simulink library "ayazLiftingBody_cl"  (R2018b)
settings: Solver=VariableStepAuto  StartTime=0.0  StopTime=10.0  RelTol=1e-3
undefined symbols (not defined in the file or in its folder): ini_euler_ang, ini_O_Vcm_o, ini_OwB, ini_Rcm_o
libraries: thrAttachPtKinematics_ul x3, eulAng2RotMat_ul x1
settings Model: Creator=mcobb  LastModifiedBy=mcobb

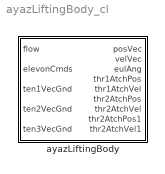
== system ayazLiftingBody_cl ==
  ayazLiftingBody : Subsystem

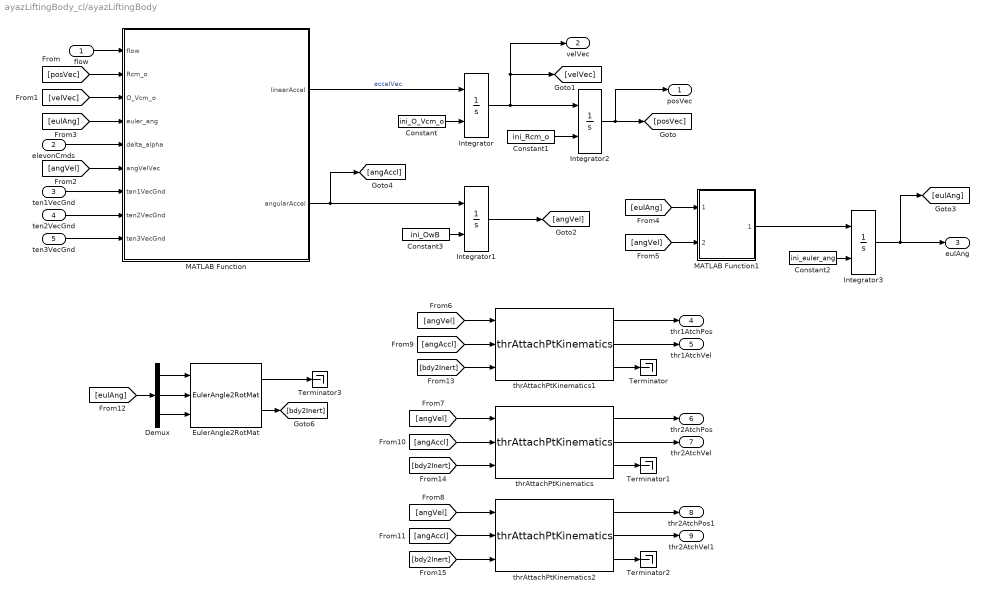
== system ayazLiftingBody_cl/ayazLiftingBody ==
  flow : Inport
  elevonCmds : Inport  Port=2
  ten1VecGnd : Inport  Port=3
  ten2VecGnd : Inport  Port=4
  ten3VecGnd : Inport  Port=5
  Constant : Constant  Value=ini_O_Vcm_o
  Constant1 : Constant  Value=ini_Rcm_o
  Constant2 : Constant  Value=ini_euler_ang
  Constant3 : Constant  Value=ini_OwB
  Demux : Demux  Outputs=3
  EulerAngle2RotMat : eulAng2RotMat_ul/EulerAngle2RotMat  SystemSampleTime=-1
  Integrator{,1..3} (4 alike) : Integrator  InitialConditionSource=external
  MATLAB Function : MATLAB Function  TreatAsAtomicUnit=on
  MATLAB Function1 : MATLAB Function  TreatAsAtomicUnit=on
  Terminator{,1..3} (4 alike) : Terminator
  thrAttachPtKinematics : thrAttachPtKinematics_ul/thrAttachPtKinematics  theAtchPosVec=sim_param.tether_imp_nodes.R2n_cm
  thrAttachPtKinematics1 : thrAttachPtKinematics_ul/thrAttachPtKinematics  theAtchPosVec=sim_param.tether_imp_nodes.R1n_cm
  thrAttachPtKinematics2 : thrAttachPtKinematics_ul/thrAttachPtKinematics  theAtchPosVec=sim_param.tether_imp_nodes.R3n_cm
  "posVec " : Outport
  velVec : Outport  Port=2
  eulAng : Outport  Port=3
  thr1AtchPos : Outport  Port=4
  thr1AtchVel : Outport  Port=5
  thr2AtchPos : Outport  Port=6
  thr2AtchVel : Outport  Port=7
  thr2AtchPos1 : Outport  Port=8
  thr2AtchVel1 : Outport  Port=9
  wires:
  ten3VecGnd/1 -> MATLAB Function/9(ten3VecGnd)
  ten2VecGnd/1 -> MATLAB Function/8(ten2VecGnd)
  ten1VecGnd/1 -> MATLAB Function/7(ten1VecGnd)
  [eulAng] -> MATLAB Function/4(euler_ang)
  [angVel] -> MATLAB Function/6(angVelVec)
  Integrator3/1 -> eulAng/1, [eulAng]
  [velVec] -> MATLAB Function/3(O_Vcm_o)
  [posVec] -> MATLAB Function/2(Rcm_o)
  Integrator2/1 -> "posVec "/1, [posVec]
  Integrator/1 -> velVec/1, [velVec], Integrator2/1
  Integrator1/1 -> [angVel]
  MATLAB Function/2(angularAccel) -> [angAccl], Integrator1/1
  MATLAB Function/1(linearAccel) -> Integrator/1  "accelVec"
  flow/1 -> MATLAB Function/1(flow)
  elevonCmds/1 -> MATLAB Function/5(delta_alpha)
  Constant/1 -> Integrator/2
  Constant1/1 -> Integrator2/2
  Constant2/1 -> Integrator3/2
  Constant3/1 -> Integrator1/2
  [eulAng] -> MATLAB Function1/1(eulAng)
  [angVel] -> MATLAB Function1/2(angVel)
  MATLAB Function1/1(eulAngDeriv) -> Integrator3/1
  [angVel] -> thrAttachPtKinematics1/1
  [angVel] -> thrAttachPtKinematics/1
  [angVel] -> thrAttachPtKinematics2/1
  [angAccl] -> thrAttachPtKinematics1/2
  [angAccl] -> thrAttachPtKinematics/2
  [angAccl] -> thrAttachPtKinematics2/2
  [eulAng] -> Demux/1
  Demux/2 -> EulerAngle2RotMat/2
  Demux/1 -> EulerAngle2RotMat/1
  Demux/3 -> EulerAngle2RotMat/3
  EulerAngle2RotMat/2 -> [bdy2Inert]
  [bdy2Inert] -> thrAttachPtKinematics1/3
  [bdy2Inert] -> thrAttachPtKinematics/3
  [bdy2Inert] -> thrAttachPtKinematics2/3
  thrAttachPtKinematics1/1 -> thr1AtchPos/1
  thrAttachPtKinematics/1 -> thr2AtchPos/1
  thrAttachPtKinematics2/1 -> thr2AtchPos1/1
  thrAttachPtKinematics1/2 -> thr1AtchVel/1
  thrAttachPtKinematics/2 -> thr2AtchVel/1
  thrAttachPtKinematics1/3 -> Terminator/1
  thrAttachPtKinematics/3 -> Terminator1/1
  thrAttachPtKinematics2/2 -> thr2AtchVel1/1
  thrAttachPtKinematics2/3 -> Terminator2/1
  EulerAngle2RotMat/1 -> Terminator3/1

== matlab function ayazLiftingBody_cl/ayazLiftingBody/MATLAB Function ==
  data: sim_param parameter; flow input; linearAccel output size=[3 1]; Rcm_o input; O_Vcm_o input; euler_ang input; delta_alpha input; angVelVec input; angularAccel output size=[3 1]; ten1VecGnd input; ten2VecGnd input; ten3VecGnd input
function [linearAccel, angularAccel] = B_F_and_T_aero(sim_param,flow,Rcm_o,...
    O_Vcm_o,euler_ang,delta_alpha,angVelVec,ten1VecGnd,ten2VecGnd,...
    ten3VecGnd)

% %% extract from structure
% aero_param = sim_param.aero_param;
% env_param = sim_param.env_param;
% turbine_param = sim_param.turbine_param;
% elevons_param = sim_param.elevons_param;
% 
% CM_nom = elevons_param.CM_nom;
% k_CM = elevons_param.k_CM;
% 
% MI = sim_param.geom_param.MI;
% Ixx = MI(1,1);
% Iyy = MI(2,2);
% Izz = MI(3,3);
% Izz_added = sim_param.geom_param.Izz_added;
% 
% Rcb_cm = sim_param.geom_param.center_of_buoy;
% 
% R1n_cm = sim_param.tether_imp_nodes.R1n_cm;
% R2n_cm = sim_param.tether_imp_nodes.R2n_cm;
% R3n_cm = sim_param.tether_imp_nodes.R3n_cm;
% 
% % buoyancy force in the ko direction
% fz_buoy = sim_param.geom_param.F_buoy;
% 
% % buoyancy force in the O frame
% O_F_buoy = [0;0;fz_buoy];
% 
% 
% % R11_g = sim_param.tether_imp_nodes.R11_g;
% % R21_g = sim_param.tether_imp_nodes.R21_g;
% % R31_g = sim_param.tether_imp_nodes.R31_g;
% 
m = sim_param.geom_param.mass;
m_added = sim_param.geom_param.m_added;
% 
% rho = env_param.density;
% 
% span = sim_param.geom_param.span;
% chord = sim_param.geom_param.chord;
% AR = sim_param.geom_param.AR;
% Rmidspan_cm = [0;span/4;0];
% 
% Sref = aero_param.Sref;
% 
% pcl_mw = aero_param.pcl_mw;
% pcd_mw = aero_param.pcd_mw;
% pcm_mw = aero_param.pcm_mw;
% 
% HS_Sref = aero_param.HS_Sref;
% VS_Sref = aero_param.VS_Sref;
% pcl_VS = aero_param.pcl_VS;
% pcd_VS = aero_param.pcd_VS;
% pcm_VS = aero_param.pcm_VS;
% 
% A_turbine = turbine_param.A_turbine;
% CD_turb = turbine_param.CD_turb;
% Cp_turb = turbine_param.Cp_turb;
% 
% % position vectors
% Rac_cm = sim_param.geom_param.aero_center;
% Rvs_cm = aero_param.Rvs_cm;
% R1turb_cm = turbine_param.R1turb_cm;
% R2turb_cm = turbine_param.R2turb_cm;
% 
% % change in effective angle of attack due to control surfaces
% delta_alp1 = delta_alpha(1);
% delta_alp2 = delta_alpha(2);
% 
% % delta elevator control
% delta_pitch = (1/2)*(delta_alp1 + delta_alp2);
% delta_roll = delta_alp1 - delta_alp2;
% 
% % rotation matrix
% [oCb,bCo] = rotation_sequence(euler_ang);
% 
% % relative velocity in O frame
% O_Vrel = flow - O_Vcm_o;
% 
% % relative/apparent velocity in the B frame
% B_Vrel = bCo*O_Vrel;
% 
% % breaking down the relative velocity in the B frame
% vxb = B_Vrel(1); vyb = B_Vrel(2); vzb = B_Vrel(3);
% 
% % apparent flow velocity in the XZ plane
% V_app_xz = sqrt(vxb^2 + vzb^2);
% 
% % apparent flow velocity in the Xy plane
% V_app_xy = sqrt(vxb^2 + vyb^2);
% 
% % angle of attack and side slip angle
% alpha = atan2(vzb,vxb);
% beta = asin(vyb/norm(B_Vrel));
% 
% % converting to degree
% alpha_deg = alpha*(180/pi);
% beta_deg = beta*(180/pi);
% 
% %% IMPORTANT
% % limiting alpha values
% if norm(alpha_deg) > 29
%     CL_mw = polyval(pcl_mw,29);
%     CD_mw = polyval(pcd_mw,29) + CL_mw^2/(pi*AR);
%     CM_mw = polyval(pcm_mw,alpha_deg);
%     
% else
%     CL_mw = polyval(pcl_mw,alpha_deg);
%     CD_mw = polyval(pcd_mw,alpha_deg) + CL_mw^2/(pi*AR);
%     CM_mw = polyval(pcm_mw,alpha_deg);
%     
% end
% 
% % limiting beta values
% if norm(beta_deg) > 29
%     
%     CL_VS = polyval(pcl_VS,29);
%     CD_VS = polyval(pcd_VS,29);
%     CM_VS = polyval(pcm_VS,beta_deg);
%     
% else
%     CL_VS = polyval(pcl_VS,beta_deg);
%     CD_VS = polyval(pcd_VS,beta_deg);
%     CM_VS = polyval(pcm_VS,beta_deg);
%     
% end
% 
% %% MAIN WING FORCES
% % dynamic pressure
% dyn_press = (1/2)*rho*norm(B_Vrel)^2;
% 
% % wing force
% Fd_mw_app = CD_mw*dyn_press*Sref;
% Fl_mw_app = CL_mw*dyn_press*Sref;
% 
% % HS force
% Fd_hs_app = CD_mw*dyn_press*HS_Sref;
% Fl_hs_app = CL_mw*dyn_press*HS_Sref;
% 
% % drag direction
% mw_drag_dir = B_Vrel/norm(B_Vrel);
% 
% % lift direction
% mw_lz = sqrt(1/(1 + (vzb/vxb)^2));
% mw_lx = -mw_lz*(vzb/vxb);
% mw_lift_dir = [mw_lx;0;mw_lz];
% 
% % aerodynamic forces on main wing in the body frame
% B_F_drag_mw = (Fd_mw_app + Fd_hs_app)*mw_drag_dir;
% B_F_lift_mw = (Fl_mw_app + Fl_hs_app)*mw_lift_dir;
% 
% B_F_aero_mw = B_F_drag_mw + B_F_lift_mw;
% 
% %% VERTICAL STABILIZER FORCES
% % aerodynamic forces in the apparent flow frame
% Fd_VS_app = CD_VS*dyn_press*VS_Sref;
% Fl_VS_app = CL_VS*dyn_press*VS_Sref;
% 
% % lift direction
% vs_ly = sqrt(1/(1 + (vyb/vxb)^2));
% vs_lx = -vs_ly*(vyb/vxb);
% vs_lift_dir = [vs_lx;vs_ly;0];
% 
% % aerodynamic forces on rudder in the body frame
% B_F_drag_VS = Fd_VS_app*mw_drag_dir;
% B_F_lift_VS = Fl_VS_app*vs_lift_dir;
% 
% B_F_aero_VS = B_F_drag_VS + B_F_lift_VS;
% 
% %% TURBINE FORCES
% 
% Fd_turb1 = CD_turb*dyn_press*A_turbine;
% Fd_turb2 = CD_turb*dyn_press*A_turbine;
% 
% B_F_turb1 = Fd_turb1*mw_drag_dir;
% B_F_turb2 = Fd_turb2*mw_drag_dir;
% 
% gen_power = 2*0.5*rho*(vxb^3)*Cp_turb*A_turbine;
% 
% if gen_power < 0
%     gen_power = 0;
% elseif norm(gen_power) > turbine_param.rated_power
%     gen_power = turbine_param.rated_power;
% end
% 
% %% TORQUES
% % torque about roll axis due to aileron
% T_roll = [(CM_nom*k_CM*delta_roll)*dyn_press*Sref*chord;0;0];
% 
% % torque about pitch axis due to aileron
% T_pitch = [0;(CM_nom*k_CM*delta_pitch)*dyn_press*Sref*chord;0];
% 
% % torque due to aero forces on main wing about CM in the B frame
% B_T_aero_mw = cross(Rac_cm,B_F_aero_mw) + T_roll + T_pitch;
% 
% % torque due to aero forces on main wing about CM in the B frame
% B_T_aero_VS = cross(Rvs_cm,B_F_aero_VS);
% 
% % torque due to turbine drag
% B_T_aero_turb = cross(R1turb_cm,B_F_turb1) + cross(R2turb_cm,B_F_turb2);
% 
% B_F_aero = B_F_turb1 + B_F_turb2 + B_F_drag_VS + B_F_lift_VS + Fd_VS_app + Fl_VS_app + B_F_aero_mw;
% 
% % torque due to the three tethers in the B frame
% B_Tt1 = cross(R1n_cm,(bCo*ten1VecGnd(:)));
% B_Tt2 = cross(R2n_cm,(bCo*ten2VecGnd(:)));
% B_Tt3 = cross(R3n_cm,(bCo*ten3VecGnd(:)));
% 
% F_buoy = bCo*[0;0;sim_param.geom_param.vol*sim_param.env_param.density*sim_param.env_param.grav];
% 
% % torque due to buoyancy about CM in the B frame
% B_T_buoy = cross(Rcb_cm,(bCo*O_F_buoy));
% 
% % torque due to gravity about CM
% B_T_grav = [0;0;0];
% 
% F_grav = [0;0;-m*sim_param.env_param.grav];
% 
% B_F_Net = B_F_aero + F_grav + F_buoy + bCo*ten1VecGnd(:) + bCo*ten2VecGnd(:) + bCo*ten3VecGnd(:);
% 
% 
% mass_matrix = [1/(m+m_added(1)) 0 0;0 1/(m+m_added(2)) 0;0 0 1/(m+m_added(3))];
%% extracting values from sim parameters structure
N = sim_param.N;

env_param = sim_param.env_param;
geom_param = sim_param.geom_param;
aero_param = sim_param.aero_param;
turbine_param = sim_param.turbine_param;
tether_param = sim_param.tether_param;
tether_imp_nodes = sim_param.tether_imp_nodes;


m = geom_param.mass;
g = env_param.grav;
rho = env_param.density;

CD_cylinder = tether_param.CD_cylinder;
tether_youngs = tether_param.tether_youngs;


Rcb_cm = geom_param.center_of_buoy;
Rac_cm = geom_param.aero_center;
R1turb_cm = turbine_param.R1turb_cm;
R2turb_cm = turbine_param.R2turb_cm;


Rvs_cm = aero_param.Rvs_cm;

R1n_cm = tether_imp_nodes.R1n_cm;
R2n_cm = tether_imp_nodes.R2n_cm;
R3n_cm = tether_imp_nodes.R3n_cm;

R11_g = tether_imp_nodes.R11_g;
R21_g = tether_imp_nodes.R21_g;
R31_g = tether_imp_nodes.R31_g;


% calculate tether masses and spring stiffness
tether_density = tether_param.tether_density;
tether_dia = tether_param.tether_diameter;
zeta = tether_param.damping_ratio;

% tether_masses = ((tether_density*(pi/4)).*tether_dia.^2).*unstretched_l;

%% spring stiffness
% tether_CS = (pi/4)*tether_dia.^2;
% 
% full_length_stiff = tether_youngs*(tether_CS.*[1/unstretched_l(1);1/unstretched_l(2);1/unstretched_l(3)]);
% 
% ks1 = full_length_stiff(1)*(N-1);
% ks2 = full_length_stiff(2)*(N-1);
% ks3 = full_length_stiff(3)*(N-1);

%% damping coeff
% full length damping coeff
% full_length_d_coeff = zeta*(2*sqrt(full_length_stiff*m));

% tether damping coeff
% damping_coeff = full_length_d_coeff*(N-1);

% c1 = damping_coeff(1);
% c2 = damping_coeff(2);
% c3 = damping_coeff(3);


%% rotations
[oCb,bCo] = rotation_sequence(euler_ang);
% platform
% pCo = [cos(plat_ang) sin(plat_ang) 0; -sin(plat_ang) cos(plat_ang) 0; 0 0 1];
% oCp = pCo';


% L1 = unstretched_l(1);
% L2 = unstretched_l(2);
% L3 = unstretched_l(3);
% 
% L1i = L1/(N-1);
% L2i = L2/(N-1);
% L3i = L3/(N-1);


%% force calculations
% buoyancy force in the ko direction
fz_buoy = geom_param.F_buoy;

% buoyancy force in the O frame
O_F_buoy = [0;0;fz_buoy];

% gravity force in the ko direction
fz_grav = -m*g;

% gravity force in the O frame
O_F_grav = [0;0;fz_grav];

% calculate aerodynamic forces on the lifting body
aero_F = B_F_and_T_aero(sim_param,flow,Rcm_o,O_Vcm_o,euler_ang,delta_alpha);

B_F_aero_mw = aero_F.B_F_aero_mw;
B_F_aero_VS = aero_F.B_F_aero_VS;
B_F_turb1 = aero_F.B_F_turb1;
B_F_turb2 = aero_F.B_F_turb2;

B_T_aero_mw = aero_F.B_T_aero_mw;
B_T_aero_VS = aero_F.B_T_aero_VS;
B_T_aero_turb = aero_F.B_T_aero_turb;


O_F_aero_mw = oCb*B_F_aero_mw;
O_F_aero_VS = oCb*B_F_aero_VS;
O_F_turb1 = oCb*B_F_turb1;
O_F_turb2 = oCb*B_F_turb2;

% %% forces acting on the center of mass
O_F_ext = O_F_buoy + O_F_grav + O_F_aero_mw + O_F_aero_VS + O_F_turb1 + O_F_turb2 +...
    ten1VecGnd + ten2VecGnd + ten3VecGnd;

mass_matrix = [1/(m+m_added(1)) 0 0;0 1/(m+m_added(2)) 0;0 0 1/(m+m_added(3))];


linearAccel = oCb*(mass_matrix*bCo*O_F_ext);
B_T_buoy = cross(Rcb_cm,(bCo*O_F_buoy));
% torque due to gravity about CM
B_T_grav = [0;0;0];


% torque due to the three tethers in the B frame
B_Tt1 = cross(R1n_cm,(bCo*ten1VecGnd));
B_Tt2 = cross(R2n_cm,(bCo*ten2VecGnd));
B_Tt3 = cross(R3n_cm,(bCo*ten3VecGnd));

B_T_ext = B_T_buoy + B_T_grav + B_T_aero_mw + B_T_aero_VS + B_T_aero_turb + ...
    B_Tt1 + B_Tt2 + B_Tt3;

Tx = B_T_ext(1);
Ty = B_T_ext(2);
Tz = B_T_ext(3);

wx = angVelVec(1);
wy = angVelVec(2);
wz = angVelVec(3);

MI = sim_param.geom_param.MI;
Ixx = MI(1,1);
Iyy = MI(2,2);
Izz = MI(3,3);
Izz_added = sim_param.geom_param.Izz_added;

angularAccel = [...
    (1/Ixx)*(Tx + (Iyy - Izz)*wy*wz);...
    (1/Iyy)*(Ty + (Izz - Ixx)*wx*wz);...
    (1/(Izz+Izz_added))*(Tz + (Ixx - Iyy)*wx*wy)];

end

== matlab function ayazLiftingBody_cl/ayazLiftingBody/MATLAB Function1 ==
  data: eulAng input; eulAngDeriv output; angVel input
function eulAngDeriv = fcn(eulAng,angVel)

wx = angVel(1);
wy = angVel(2);
wz = angVel(3);

ph = eulAng(1);
th = eulAng(2);

eulAngDeriv = zeros(3,1);
eulAngDeriv(1) = wx + sin(ph)*tan(th)*wy + cos(ph)*tan(th)*wz;
eulAngDeriv(2) = cos(ph)*wy - sin(ph)*wz;
eulAngDeriv(3) = sec(th)*sin(ph)*wy + cos(ph)*sec(th)*wz;
